simulink model "SemiOffline_DataImport_AND_Preprocessing_ECGandSCG3D"  (R2019a)
settings: Solver=FixedStepDiscrete  StartTime=0.0  StopTime=sim_time + param_frame_size_sec  FixedStep=1/fs  MaxStep=1/fs  RelTol=1e-3
undefined symbols (not defined in the file): fdesignblkfcn, fs, gcbh, param_frame_size_sec, tot_samples
(part 3 of 3)

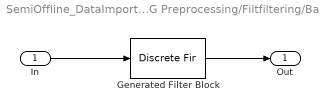
== system SemiOffline_DataImport_AND_Preprocessing_ECGandSCG3D/SCG Preprocessing/Filtfiltering/Bandpass Filter 2 ==
  In : Inport
  Generated Filter Block : DiscreteFir  Tag=BlockMethodSubSystem  Coefficients=[-0.000647770338075434929 -0.000343517502483878777 -0.000420326780186868994 -0.000497874681447326448 -0.000572163883567983742 -0.000640228248060424696 -0.000697341620736447246 -0.000741100378547245487 -0.000767502343489427749 -0.000773945311594367771 -0.000756163673465519263 -0.000715781040457746714 -0.000649518851291922667 -0.000558754413187999722 -0.00044468802672256876 -0.000309569390145499881 -0.000157346999555588955 7.56309344158924597e-06 0.00017981999696271481 0.000352907358331129323 0.000520173062377952814 0.000675059629141158213 0.000810832524492023751 0.000920902297954280416 0.00100022555744028814 0.00104339585916609994 0.00104784075236300563 0.00101082276479851942 0.000932493196038372985 0.00081372483012750324 0.000658118786716569456 0.000469697822827719303 0.000255159625340334827 2.14396010500159063e-05 -0.000222748792724650451 -0.000468614551614006489 -0.000706670354182749056 -0.000927970460822908987 -0.00112339311178654235 -0.00128559051618629583 -0.0014075719529827971 -0.0014847378077428345 -0.00151343561916275301 -0.00149285314374439848 -0.00142321603360264838 -0.00130784430924640264 -0.0011507255600504238 -0.000958682411888284636 -0.000738927946466580573 -0.000500553073942569017 -0.000252448107042536841 -4.51228298674853645e-06 0.000234444470312946134 0.000455461207387870327 0.000651469166657359794 0.000816082599625653801 0.000945275154119637169 0.00103619033374766209 0.00108877327251135801 0.00110401335657345613 0.00108571053871140614 0.00103834647166455344 0.000968694804841021824 0.000883612324176489129 0.00079141959854462133 0.000699633357995322258 0.000616426848716069425 0.000548300984414140311 0.000501481625634690124 0.000479961455332933733 0.000486789456532214109 0.000522442357222020651 0.00058627283270533989 0.000674998416817543592 0.000784500194055535245 0.000908445013836128119 0.00104019836345509912 0.00117163853730648101 0.00129524246150523035 0.00140281134401658617 0.00148771616471947161 0.00154348036758589994 0.00156593860019076754 0.00155180420574065276 0.00150047956618671327 0.0014125221351874741 0.00129124537708533681 0.00114095226621692479 0.000968283947858580374 0.000780347697060279968 0.00058580174682495306 0.000392949669008726315 0.000210739838125063969 4.67353233640661067e-05 -9.17098537984661032e-05 -0.000199474799964817527 -0.000272369167151098905 -0.000308956715154304199 -0.000309062680725871372 -0.000275382856037888104 -0.000211718414908937836 -0.00012440394301087011 -2.03462178716174195e-05 9.18365595282383371e-05 0.000203774330319042617 0.000306382694897032286 0.00039183217102360077 0.000452554892511169168 0.000483155558882161773 0.000479279720088677912 0.000439316668050006678 0.000363105403623313172 0.000253394761208263191 0.000114230004232997954 -4.77446668554886442e-05 -0.000225181088213468402 -0.000408917488377553637 -0.000589991911142579025 -0.00075869987196111393 -0.000906593394805637102 -0.00102553663011526602 -0.00110963698146597858 -0.00115418825375746253 -0.00115734164105921774 -0.00111890913599901019 -0.00104171557147943856 -0.000930164097664520385 -0.000791336524032147009 -0.000633259801675410032 -0.000465832430360793397 -0.000298919925422787205 -0.000143130722921475659 -7.86877071387343148e-06 9.78644949485511892e-05 0.000167363222362294718 0.00019525861251619436 0.000179203991855867199 0.000118725167489869548 1.6541729219412952e-05 -0.000122793742983712804 -0.000291899772648228362 -0.000482194263276236991 -0.000683150339584172187 -0.00088409319788581046 -0.00107362450916950779 -0.00124144751215223763 -0.00137781033119710916 -0.00147526394058089061 -0.00152791278658659293 -0.00153299420877785588 -0.00148987526532067937 -0.00140130121930216343 -0.00127211455353073055 -0.00111015084855621581 -0.000924679192769932478 -0.000727023678111190933 -0.000528801782353420513 -0.000342348805686419622 -0.00017894991212643208 -4.92046497649435222e-05 3.86290643596606527e-05 7.81216788691107265e-05 6.61062040557425386e-05 1.87789399799218092e-06 -0.000111703526733958531 ...(+15232 chars)]  InputProcessing=Columns as channels (frame based)
  Out : Outport
  wires:
  In/1 -> Generated Filter Block/1
  Generated Filter Block/1 -> Out/1
